simulink model "sldemo_zeroxing"  (Simulink 10.0)
settings: Solver=VariableStepDiscrete  StartTime=0.0  StopTime=10  RelTol=1e-3  AbsTol=1e-6
StartFcn:
  | set_param('sldemo_zeroxing/Scope','Open','on')
Description:
  | Accurate Zero-Crossing Detection
  | 
  | This example shows how zero crossings work in Simulink(R).
  | In this model, three shifted sine waves are fed into an absolute value
  | block and saturation block. At exactly t = 5, the output of the switch block
  | changes from the absolute value to the saturation block. Zero crossings
  | in Simulink will automatically detect exactly when the switch block
  | changes its output, and the solver will step to the exact time that the
  | event happens. This can be seen by examining the output in the scope.
settings Model: Creator=The MathWorks, Inc.  LastModifiedBy=bhisma  ExtModeTrigMode=oneshot  ExtModeAutoUpdateStatusClock=off
settings SolverCC: AutoScaleAbsTol=off
settings DataIOCC: ExternalInput=[]  InitialState=[]  SaveOutput=off  SaveTime=off  ReturnWorkspaceOutputs=on
settings OptimizationCC: BlockReduction=off  BooleanDataType=off  InitFltsAndDblsToZero=on  BufferReusableBoundary=off
settings DebuggingCC: SaveWithParameterizedLinksMsg=none  SignalResolutionControl=TryResolveAllWithWarning  MultiTaskDSMMsg=warning  MultiTaskCondExecSysMsg=none  FcnCallInpInsideContextMsg=warning  BusObjectLabelMismatch=none
settings HardwareCC: TargetUnknown=on
settings GRTTargetCC: TargetFcnLib=ansi_tfl_tmw.mat  GeneratePreprocessorConditionals=Disable all
settings ConfigComp: CovMetricSettings=d  CovExternalEMLEnable=off

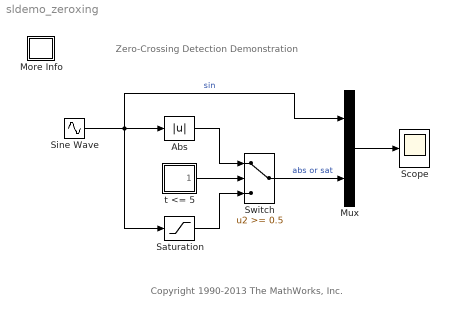
== system sldemo_zeroxing ==
  note: Zero-Crossing Detection Demonstration
  note: Copyright 1990-2013 The MathWorks, Inc.
  Abs : Abs  SaturateOnIntegerOverflow=on
  More Info : Subsystem
      settings: OpenFcn=showExample('simulink_general/sldemo_zeroxingExample')
      mask Display: disp('?')
  Mux : Mux  Inputs=2
  Saturation : Saturate  UpperLimit=[0.5 .55 .6]  LowerLimit=[-0.5 -.55 -.6]
  Scope : Scope
  Sine Wave : Sin  Phase=[.1 .2 .3]  SampleTime=0
  Switch : Switch  Threshold=0.5  SaturateOnIntegerOverflow=on  InputSameDT=on
  t <= 5 : Subsystem
  wires:
  t <= 5/1(t <= 5) -> Switch/2
  Switch/1 -> Mux/2  "abs or sat"
  Saturation/1 -> Switch/3
  Abs/1 -> Switch/1
  Sine Wave/1 -> Abs/1, Mux/1, Saturation/1  "sin"
  Mux/1 -> Scope/1

== system sldemo_zeroxing/More Info ==

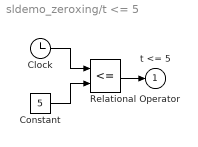
== system sldemo_zeroxing/t <= 5 ==
  Clock : Clock
  Constant : Constant  Value=5
  Relational Operator : RelationalOperator  Operator=<=  RndMeth=Nearest  InputSameDT=on
  t <= 5 : Outport  InitialOutput=0  VectorParamsAs1DForOutWhenUnconnected=off
  wires:
  Constant/1 -> Relational Operator/2
  Clock/1 -> Relational Operator/1
  Relational Operator/1 -> t <= 5/1
